simulink model "Waehrungsmodelle"  (R2014a)
settings: Solver=ode1  StartTime=0.0  StopTime=100  FixedStep=1  MaxStep=1  MinStep=1  RelTol=1e-3
(part 16 of 18)

== system Waehrungsmodelle/Währungssystem6/Populationsmodell ==
  note: Geburten
  Umweltqualität : Inport
  Dienstleistungsqualität : Inport  Port=2
  Güterangebotsqualität bei vorhandem Einkommen : Inport  Port=3
  Ausgleichsfaktor : Constant  Value=0.3
  Dienstleistungs- multiplikator : Sum
  Divide1 : Product  Inputs=*/
  Divide2 : Product  Inputs=*/
  Divide3 : Product  Inputs=*/
  Erwachsene : Sum  Inputs=+--
  Fertilitätsmultiplikator : Product  Inputs=4
  Fertilitätsrate pro Frau : Constant  Value=3/40
  Frauenanteil pro Erwachsene : Constant  Value=0.5
  Güterangebotsqualitäts- multiplikator : Sum
  Jahre der Altersklasse : Constant  Value=15
  Jahre der Altersklasse1 : Constant  Value=10
  Jahre der Altersklasse2 : Constant  Value=40
  Kinder : Sum  Inputs=+--
  Lebensqualitätsfaktor : Product  Inputs=/
  Product{,1..3} (4 alike) : Product  Inputs=3
  Schüler / Studenten : Sum  Inputs=+--
  Start Erwachsene: 55 : Integrator  InitialCondition=55
  Start Kinder: 13 : Integrator  InitialCondition=13
  Start Schüler: 11 : Integrator  InitialCondition=11
  Sterblichkeitsrate Kinder : Constant  Value=0.003
  Sterblichkeitsrate1 : Constant  Value=0.002
  Sterblichkeitsrate2 : Constant  Value=0.004
  Umwelt- multiplikator : Sum
  Erwerbsfähige : Outport
  wires:
  Product/1 -> Kinder/1
  Jahre der Altersklasse2/1 -> Divide3/2
  Jahre der Altersklasse/1 -> Divide1/2
  Divide1/1 -> Schüler / Studenten/1, Kinder/3
  Sterblichkeitsrate1/1 -> Product1/2
  Sterblichkeitsrate Kinder/1 -> Product2/2
  Divide2/1 -> Schüler / Studenten/3, Erwachsene/1
  Start Schüler: 11/1 -> Product1/3, Divide2/1
  Jahre der Altersklasse1/1 -> Divide2/2
  Sterblichkeitsrate2/1 -> Product3/2
  Start Erwachsene: 55/1 -> Erwerbsfähige/1, Product3/3, Divide3/1, Product/1
  Erwachsene/1 -> Start Erwachsene: 55/1
  Kinder/1 -> Start Kinder: 13/1
  Start Kinder: 13/1 -> Product2/3, Divide1/1
  Schüler / Studenten/1 -> Start Schüler: 11/1
  Ausgleichsfaktor/1 -> Umwelt- multiplikator/2, Güterangebotsqualitäts- multiplikator/1, Dienstleistungs- multiplikator/1
  Fertilitätsmultiplikator/1 -> Product/3
  Umweltqualität/1 -> Umwelt- multiplikator/1
  Dienstleistungs- multiplikator/1 -> Lebensqualitätsfaktor/1, Fertilitätsmultiplikator/4
  Fertilitätsrate pro Frau/1 -> Fertilitätsmultiplikator/1
  Umwelt- multiplikator/1 -> Fertilitätsmultiplikator/2
  Dienstleistungsqualität/1 -> Dienstleistungs- multiplikator/2
  Product2/1 -> Kinder/2
  Product1/1 -> Schüler / Studenten/2
  Divide3/1 -> Erwachsene/3
  Product3/1 -> Erwachsene/2
  Lebensqualitätsfaktor/1 -> Product3/1, Product1/1, Product2/1
  Güterangebotsqualität bei vorhandem Einkommen/1 -> Güterangebotsqualitäts- multiplikator/2
  Güterangebotsqualitäts- multiplikator/1 -> Fertilitätsmultiplikator/3
  Frauenanteil pro Erwachsene/1 -> Product/2

== system Waehrungsmodelle/Währungssystem6/Staat ==
  Kreditvergabe : Inport
  Kreditrückzahlung : Inport  Port=2
  Finanzbedarf Arbeitslosigkeit : Inport  Port=3
  Dienstleistungsqualität : Inport  Port=4
  Steuern Bank : Inport  Port=5
  Steuern Unternehmen : Inport  Port=6
  Rohstoffabgabe : Inport  Port=7
  Umweltqualität : Inport  Port=8
  MATLAB Function : MATLAB Function  TreatAsAtomicUnit=on
  Kreditbedarf : Outport
  Finanzierung Öffentlicher Dienstleistungen : Outport  Port=2
  Geldbestand Staat : Outport  Port=3
  Steuersatz : Outport  Port=4
  Ressourcen Steuer : Outport  Port=5
  wires:
  Steuern Unternehmen/1 -> MATLAB Function/6(SteuernUnternehmen)
  Dienstleistungsqualität/1 -> MATLAB Function/4(Dienstleistungsqualitaet)
  MATLAB Function/4(SteuersatzOut) -> Steuersatz/1
  MATLAB Function/2(FinanzierungOeffentlicheDienstleistungen) -> Finanzierung Öffentlicher Dienstleistungen/1
  Finanzbedarf Arbeitslosigkeit/1 -> MATLAB Function/3(FinanzbedarfArbeitslosigkeit)
  MATLAB Function/3(GeldbestandStaat) -> Geldbestand Staat/1
  Kreditrückzahlung/1 -> MATLAB Function/2(Kreditrueckzahlung)
  MATLAB Function/1(Kreditbedarf) -> Kreditbedarf/1
  Steuern Bank/1 -> MATLAB Function/5(SteuernBanken)
  Kreditvergabe/1 -> MATLAB Function/1(KreditvergabeNeuStaat)
  MATLAB Function/5(RessourcenAbgabesatzOut) -> Ressourcen Steuer/1
  Rohstoffabgabe/1 -> MATLAB Function/7(Rohstoffabgabe)
  Umweltqualität/1 -> MATLAB Function/8(Umweltqualitaet)

== system Waehrungsmodelle/Währungssystem6/Umwelt ==
  Ressourcenbedarf : Inport
  Umwelt : MATLAB Function  TreatAsAtomicUnit=on
  abgebaute Ressourcen : Outport
  verhandene Ressourcen : Outport  Port=2
  Umweltqualität : Outport  Port=3
  wires:
  Umwelt/3(Umweltqualitaet) -> Umweltqualität/1
  Umwelt/2(VorhandeneRessourcenOut) -> verhandene Ressourcen/1
  Umwelt/1(AbgebauteRessourcen) -> abgebaute Ressourcen/1
  Ressourcenbedarf/1 -> Umwelt/1(Ressourcenbedarf)

== system Waehrungsmodelle/Währungssystem6/Unternehmen ==
  Erwerbsfähige : Inport
  Neue Kreditvergabe der Unternehmen : Inport  Port=2
  Kreditrückzahlung der Unternehmen : Inport  Port=3
  Rohstoffe : Inport  Port=4
  Güterkonsum Inland : Inport  Port=5
  Güterkonsum Ausland : Inport  Port=6
  RessourcenAbgabe Steuersatz : Inport  Port=7
  Kreditzinssatz Inland : Inport  Port=8
  Kreditzinssatz Ausland : Inport  Port=9
  Steuersatz : Inport  Port=10
  Neue Kreditvergabe der Unternehmen Ausland : Inport  Port=11
  Kreditrückzahlung der Unternehmen Ausland : Inport  Port=12
  MATLAB Function : MATLAB Function  TreatAsAtomicUnit=on
  Inflation : Outport
  Rohstoffbedarf : Outport  Port=2
  Arbeitsplätze der Unternehmen : Outport  Port=3
  Güterangebot Inland : Outport  Port=4
  Arbeitslohn : Outport  Port=5
  zukünftiger Arbeitsdarf der Unternehmen : Outport  Port=6
  Güterpreis : Outport  Port=7
  Steuern von Unternehmen : Outport  Port=8
  Rohstoffabgabe : Outport  Port=9
  Kreditbedarf Inland : Outport  Port=10
  Kreditbedarf Ausland : Outport  Port=11
  Technischer Fortschritt Rationalität : Outport  Port=12
  Technischer Fortschritt Ressourcen : Outport  Port=13
  Wirtschaftswachstum : Outport  Port=14
  Güterangebot Ausland : Outport  Port=15
  wires:
  MATLAB Function/8(SteuernUnternehmen) -> Steuern von Unternehmen/1
  MATLAB Function/7(GueterpreisOut) -> Güterpreis/1
  Neue Kreditvergabe der Unternehmen/1 -> MATLAB Function/2(NeueKreditvergabeUnternehmen)
  Kreditrückzahlung der Unternehmen/1 -> MATLAB Function/3(KreditrueckzahlungUnternehmen)
  MATLAB Function/6(BenoetigterArbeitsbedarfUnternehmen) -> zukünftiger Arbeitsdarf der Unternehmen/1
  MATLAB Function/4(GueterangebotInland) -> Güterangebot Inland/1
  MATLAB Function/5(ArbeitslohnOut) -> Arbeitslohn/1
  MATLAB Function/2(Rohstoffbedarf) -> Rohstoffbedarf/1
  MATLAB Function/1(Inflation) -> Inflation/1
  Erwerbsfähige/1 -> MATLAB Function/1(Erwerbsfaehige)
  MATLAB Function/3(ArbeitsplaetzeUnternehmen) -> Arbeitsplätze der Unternehmen/1
  Rohstoffe/1 -> MATLAB Function/4(Rohstoffe)
  Güterkonsum Inland/1 -> MATLAB Function/5(GueterkonsumInland)
  MATLAB Function/9(RessourcenAbgabeSteuer) -> Rohstoffabgabe/1
  MATLAB Function/11(KreditbedarfAusland) -> Kreditbedarf Ausland/1
  MATLAB Function/12(TechnischeVerbesserungRationalitaetOut) -> Technischer Fortschritt Rationalität/1
  MATLAB Function/13(TechnischeVerbesserungRessourcenOut) -> Technischer Fortschritt Ressourcen/1
  Güterkonsum Ausland/1 -> MATLAB Function/6(GueterkonsumAusland)
  RessourcenAbgabe Steuersatz/1 -> MATLAB Function/7(RessourcenAbgabeSteuersatz)
  Kreditzinssatz Inland/1 -> MATLAB Function/8(KreditZinssatzInland)
  Kreditzinssatz Ausland/1 -> MATLAB Function/9(KreditZinssatzAusland)
  Steuersatz/1 -> MATLAB Function/10(Steuersatz)
  MATLAB Function/10(KreditbedarfInland) -> Kreditbedarf Inland/1
  MATLAB Function/14(Wirtschaftswachstum) -> Wirtschaftswachstum/1
  MATLAB Function/15(GueterangebotAusland) -> Güterangebot Ausland/1
  Neue Kreditvergabe der Unternehmen Ausland/1 -> MATLAB Function/11(NeueKreditvergabeUnternehmenAusland)
  Kreditrückzahlung der Unternehmen Ausland/1 -> MATLAB Function/12(KreditrueckzahlungUnternehmenAusland)

== system Waehrungsmodelle/Währungssystem6/Wechselkursberechnung ==
  Güterpreis Ausland : Inport
  Güterkonsum im Inland von Gütern vom Ausland : Inport  Port=2
  Güterkonsum im Ausland von Gütern im Inland : Inport  Port=3
  MATLAB Function : MATLAB Function  TreatAsAtomicUnit=on
  Güterpreis Ausland in Eigenwährung : Outport
  Wechselkursfaktor : Outport  Port=2
  Gesamter Güterkonsum im Ausland von Gütern im Inland : Outport  Port=3
  Gesamter Güterkonsum im Inland von Gütern vom Ausland : Outport  Port=4
  wires:
  Güterpreis Ausland/1 -> MATLAB Function/1(GueterpreisAusland)
  Güterkonsum im Inland von Gütern vom Ausland/1 -> MATLAB Function/2(GueterKonsumImInlandVomAusland)
  Güterkonsum im Ausland von Gütern im Inland/1 -> MATLAB Function/3(GueterKonsumImAuslandVomInland)
  MATLAB Function/1(GueterpreisAuslandInEigenwaehrung) -> Güterpreis Ausland in Eigenwährung/1
  MATLAB Function/2(Wechselkursfaktor) -> Wechselkursfaktor/1
  MATLAB Function/3(GesamterGueterKonsumImAuslandVomInlandOut) -> Gesamter Güterkonsum im Ausland von Gütern im Inland/1
  MATLAB Function/4(GesamterGueterKonsumImInlandVomAuslandOut) -> Gesamter Güterkonsum im Inland von Gütern vom Ausland/1

== system Waehrungsmodelle/Währungssystem6/Öffentliche Dienstleistungen ==
  Finanzierung : Inport
  Erwerbsfähige : Inport  Port=2
  Arbeitslohn : Inport  Port=3
  MATLAB Function : MATLAB Function  TreatAsAtomicUnit=on
  Arbeitsplätze Dienstleistung : Outport
  Dienstleistungsqualität : Outport  Port=2
  wires:
  Arbeitslohn/1 -> MATLAB Function/3(Arbeitslohn)
  Erwerbsfähige/1 -> MATLAB Function/2(Erwerbsfaehige)
  Finanzierung/1 -> MATLAB Function/1(Finanzierung)
  MATLAB Function/1(ArbeitsplaetzeDienstleistung) -> Arbeitsplätze Dienstleistung/1
  MATLAB Function/2(Dienstleistungsqualitaet) -> Dienstleistungsqualität/1

== matlab function Waehrungsmodelle/Währungssystem1/Haushalte/MATLAB Function ==
  data: Erwerbsfaehige input; GueterkonsumInland output; ArbeitsplaetzeDienstleistungen input; ArbeitsplaetzeUnternehmen input; NeueKreditvergabeInland input; KreditrueckzahlungInland input; GueterAngebotInland input; Arbeitslohn input; GueterpreisInland input; FinanzierungArbeitslosigkeit output; Spareinlagen output; KreditbedarfInland output; ArbeiterUnternehmen output; GueterVorratHaushalte output; GueterangebotsqualitaetOut output; Arbeitslosenquote output; GueterpreisAusland input; GueterkonsumAusland output; KreditbedarfAusland output; NeueKreditvergabeAusland input; KreditrueckzahlungAusland input; GueterAngebotAusland input; KreditZinssatzInland input; KreditZinssatzAusland input
function [GueterkonsumInland, FinanzierungArbeitslosigkeit, Spareinlagen, KreditbedarfInland, ...
              ArbeiterUnternehmen, GueterVorratHaushalte, GueterangebotsqualitaetOut, ...
              Arbeitslosenquote, GueterkonsumAusland, KreditbedarfAusland] = ...
    Haushalte(Erwerbsfaehige, ArbeitsplaetzeDienstleistungen, ArbeitsplaetzeUnternehmen, ...
            NeueKreditvergabeInland, KreditrueckzahlungInland, GueterAngebotInland, Arbeitslohn, ...
            GueterpreisInland, GueterpreisAusland, NeueKreditvergabeAusland, ...
            KreditrueckzahlungAusland, GueterAngebotAusland, KreditZinssatzInland, KreditZinssatzAusland)
 %# Submodul zur Berechnung der Abläufe bzgl. der Haushalte
 
% Es wird eine Gütereinheit pro Zeiteinheit und Erwerbsfaehiger
% verbraucht;
persistent GueterVorrat;

% Angebotsqualität der Güter [0 - 1]
% Werden weniger Güter angeboten als benötigt oder ist die Anzahl der 
% benötigten Güter nicht mehr bezahlbar sinkt die Qualität
persistent Gueterangebotsqualitaet;

    % Anfangsvorrat
    if isempty(GueterVorrat)
       GueterVorrat = 100;
    end 
    
    if isempty(Gueterangebotsqualitaet)
       Gueterangebotsqualitaet = 1;
    end     
    
    % Beschäftigte bei Öffentlichen Dienstleistungen bekommen 80 % vom
    % Lohnniveau der Unternehmen
    Dienstleistungslohnfaktor = 0.8;
    
    % Arbeitslose bekommen vom Staat 50% des Lohnnivaus
    Arbeitslosenlohnfaktor = 0.5;    
    
    % Maximale Vorratszeit
    MaximaleVorratszeit = 4;
    
    % Der maximale Vorrat gilt für 4 Zeiteinheiten
    MaximalerVorrat = Erwerbsfaehige * MaximaleVorratszeit; 
    
    
    % Gueterverbrauch pro Zeiteinheit
    GueterVorrat = GueterVorrat -  Erwerbsfaehige;    

    if GueterVorrat <= 0
         % Sind weniger Vorräte als fuer eine Zeiteinheit vorhanden, 
         % sinkt die Güterqualität
        Gueterangebotsqualitaet = Gueterangebotsqualitaet - 0.1;
        Gueterangebotsqualitaet = max(Gueterangebotsqualitaet, 0);
    else 
         % Sind mehr Vorräte als fuer eine Zeiteinheit vorhanden, 
         % steigt die Güterqualität        
        Gueterangebotsqualitaet = Gueterangebotsqualitaet + 0.1;
        Gueterangebotsqualitaet = min(Gueterangebotsqualitaet, 1);        
    end       
    
    GueterangebotsqualitaetOut = Gueterangebotsqualitaet;  
    
    % Es können maximal die vergleibenden Erwerbsfähigen oder der
    % notwendige Arbeiterbedarf eingesetzt werden
    ArbeiterUnternehmen = Erwerbsfaehige - ArbeitsplaetzeDienstleistungen;
    
    % die Arbeitslosen sind alle Erwerbsfähigen, welche keinen Arbeitsplatz
    % haben
    Arbeitslose = Erwerbsfaehige - (ArbeitsplaetzeUnternehmen + ArbeitsplaetzeDienstleistungen );
    % Arbeitslosenquote [0 - 1]
    % Auf Grund von Rundungen kann die Arbeitslosenquote min. 0 sein.
    Arbeitslosenquote = max(0, Arbeitslose / Erwerbsfaehige);
    
   
    
    % Einkommensberechnung für die Arbeitsplätze bei Unternehmen
    EinkommenUnternehmen = ArbeitsplaetzeUnternehmen * Arbeitslohn ;
    
    % Einkommensberechnung für die Arbeitsplätze bei Öffentlichen Dienstleistungen
    EinkommenDienstleistungen = ArbeitsplaetzeDienstleistungen * Arbeitslohn * Dienstleistungslohnfaktor;
    
    % Finanzierungsbedarf fuer Arbeitslosigkeit
    EinkommenArbeitslosigkeit = Arbeitslose * Arbeitslohn * Arbeitslosenlohnfaktor;
    FinanzierungArbeitslosigkeit = EinkommenArbeitslosigkeit;
    
    % Berechnung des Gesamteinkommens
    Gesamteinkommen = EinkommenUnternehmen + EinkommenDienstleistungen + EinkommenArbeitslosigkeit;           
        
    % Genehmigung der letzten Kreditanfrage
    Gesamteinkommen = Gesamteinkommen + NeueKreditvergabeInland + NeueKreditvergabeAusland;   
    
    % Rückzahlung der offenen Kreditrate
    Gesamteinkommen = Gesamteinkommen - KreditrueckzahlungInland - KreditrueckzahlungAusland;    
    
    % Prüfen welche Güter die günstigeren sind (Inlandsgüter oder
    % Auslandsgüter)
    if GueterpreisInland <= GueterpreisAusland
        % Wenn die Güter im Inland günstiger sind
        
        % Güter nachkaufen solange das Geld reicht oder das Vorratsmaximum erreicht
        % wurde, in Abhängigkeit des Güterangebots
        MoeglicheGueternachfrage = floor(Gesamteinkommen / GueterpreisInland);      
        % Die kleinste Gueternachfrage ist immer 50% des normalen
        % Verbrauchs der Güter
        GueterkonsumInland = max(0, min(MoeglicheGueternachfrage, GueterAngebotInland));

        % Wenn genug Güter auf Vorrat Komsum auf 50% senken
        if GueterVorrat > MaximalerVorrat
            GueterkonsumInland = GueterkonsumInland / 2;    
        end

        GueterVorrat = GueterVorrat + GueterkonsumInland;
        UebrigesGueterangebot = GueterAngebotInland - GueterkonsumInland;
        UebrigesEinkommen = Gesamteinkommen - (GueterkonsumInland * GueterpreisInland);  

        % Wenn noch Geld übrig ist und genug Geld vorhanden im Ausland die
        % Güter kaufen
        if GueterVorrat < MaximalerVorrat && UebrigesEinkommen > 0
            % Güter nachkaufen solange das Geld reicht oder das Vorratsmaximum erreicht
            % wurde, in Abhängigkeit des Güterangebots
            MoeglicheGueternachfrageAusland = floor(UebrigesEinkommen / GueterpreisAusland);              
            GueterkonsumAusland = max(0, min(min(MoeglicheGueternachfrageAusland, GueterAngebotAusland), MaximalerVorrat-GueterVorrat));           
            
            GueterVorrat = GueterVorrat + GueterkonsumAusland;
            UebrigesEinkommen = UebrigesEinkommen - (GueterkonsumAusland * GueterpreisAusland);                  
        else
            GueterkonsumAusland = 0;
        end        
    else
        % Wenn die Güter im Ausland günstiger sind
        
        % Güter nachkaufen solange das Geld reicht oder das Vorratsmaximum erreicht
        % wurde, in Abhängigkeit des Güterangebots
        % Es können maximal 50% der Güter aus dem Ausland gekauft werden
        MoeglicheGueternachfrage = min(0, min(Erwerbsfaehige/2, floor(Gesamteinkommen / GueterpreisAusland)));    

        GueterkonsumAusland = max(0, min(MoeglicheGueternachfrage, GueterAngebotAusland));

        % Wenn genug Güter auf Vorrat Komsum auf 50% senken
        if GueterVorrat > MaximalerVorrat
            GueterkonsumAusland = GueterkonsumAusland / 2;    
        end

        GueterVorrat = GueterVorrat + GueterkonsumAusland;

        UebrigesEinkommen = Gesamteinkommen - (GueterkonsumAusland * GueterpreisAusland);  

        % Wenn noch Geld übrig ist und genug Geld vorhanden im Ausland die
        % Güter kaufen
        if GueterVorrat < MaximalerVorrat && UebrigesEinkommen > 0
            % Güter nachkaufen solange das Geld reicht oder das Vorratsmaximum erreicht
            % wurde, in Abhängigkeit des Güterangebots
            MoeglicheGueternachfrageInland = floor(UebrigesEinkommen / GueterpreisInland);              
            GueterkonsumInland = max(0, min(MoeglicheGueternachfrageInland, GueterAngebotInland));                       
            GueterkonsumInland = GueterkonsumInland * min(0, 1.5 - GueterVorrat / MaximalerVorrat);
            
            GueterVorrat = GueterVorrat + GueterkonsumInland;
            UebrigesGueterangebot = GueterAngebotInland - GueterkonsumInland;
            UebrigesEinkommen = UebrigesEinkommen - (GueterkonsumInland * GueterpreisInland);                  
        else
            GueterkonsumInland = 0;
            UebrigesGueterangebot = 0;
        end            
    end   
    
    
    % Prüfung ob ein Kredit notwendig ist, da noch zu wenig Güter gekauft
    % wurden und Güter vorhanden sind
    if GueterVorrat < Erwerbsfaehige *2 && UebrigesGueterangebot > 0
        % Berechnung der notwendigen Güter bis zur nächsten Zeiteinheit
        BenoetigteGueter = Erwerbsfaehige;                
                        
        % Berechnung des Kreditbedarfs
        Kreditbedarf = BenoetigteGueter * GueterpreisInland;  
        % Kreditbedarf auf In- und Ausland aufteilen
        % Der Kredit mit dem geringeren Zinssatz wird bevorzugt und 70%
        % verwendet. Der teurere Kredit wird mit 30% verwendet.
        if KreditZinssatzInland <= KreditZinssatzAusland
            KreditbedarfInland = Kreditbedarf * 0.7;
            KreditbedarfAusland = Kreditbedarf * 0.3;
        else
            KreditbedarfAusland = Kreditbedarf * 0.7;
            KreditbedarfInland = Kreditbedarf * 0.3;        
        end        
    else
        % Kein Kreditbedarf
        KreditbedarfInland = 0;        
        KreditbedarfAusland = 0;  
    end
    
    % Übriges Geld sparen
    Spareinlagen = UebrigesEinkommen;
    
    GueterVorratHaushalte = GueterVorrat;

== matlab function Waehrungsmodelle/Währungssystem1/Öffentliche Dienstleistungen/MATLAB Function ==
  data: Finanzierung input; ArbeitsplaetzeDienstleistung output; Erwerbsfaehige input; Arbeitslohn input; Dienstleistungsqualitaet output
function [ArbeitsplaetzeDienstleistung, Dienstleistungsqualitaet] = OeffentlicheDienstleistungen(Finanzierung, Erwerbsfaehige, Arbeitslohn)
%# Submodul zur Berechnung das Öffentliche Dienstleistungsmodell

    persistent Arbeitsplaetze;

    % Anfangsarbeitsplätze
    if isempty(Arbeitsplaetze)
       Arbeitsplaetze = 20;
    end 

    % Da der Arbeitslohn ein Referenzlohn der privaten Unternehmen ist wird
    % dieser angepasst und um 20 % gesenkt
    LohnNiveauOeffentlicherDienst = 0.8;
    Arbeitslohn = Arbeitslohn * LohnNiveauOeffentlicherDienst;
    
    % Es können nicht mehr Arbeitsplätze wie Erwerbsfähige vorhanden sind
    % besetzt werden
    if Erwerbsfaehige < Arbeitsplaetze
        Arbeitsplaetze = Erwerbsfaehige;
    end

    % Existiert nicht genug Geld für die öffentlichen Dientleistungen
    % werden die Arbeitsplätze an die Finanzierung vom Staat angepasst.
    if (Finanzierung < Arbeitsplaetze * Arbeitslohn)
        Arbeitsplaetze = floor(Finanzierung / Arbeitslohn);        
    end          
       
    ArbeitsplaetzeDienstleistung = Arbeitsplaetze;
    
    % Berechnet Dienstleistungsqualitaet mit min:0.2 und max:1
    % indem die Arbeitsplätze der öffentlichen Dienstleistungen durch die
    % gesamten Erwerbstätigen geteilt werden und als Ausgleichfaktor mit drei
    % multipliziert wird. Somit ist es optimal wenn min. 1/3 aller
    % Erwerbsfähigen bei den öffentlichen Dienstleistungen arbeiten
    Dienstleistungsqualitaet = max(0.2, min(1, 3 * Arbeitsplaetze / Erwerbsfaehige));

== matlab function Waehrungsmodelle/Währungssystem1/Banken/MATLAB Function ==
  data: EinlagenAenderungHaushalte input; KreditbedarfHaushalte input; KreditbedarfUnternehmen input; KreditbedarfHaushalteAusland input; KreditbedarfUnternehmenAusland input; KreditbedarfStaat input; Steuersatz input; Leitzins input; Mindestreservesatz input; MaximaleNotenbankGeldmenge input; KontoHaushalteOut output; KrediteHaushalteOut output; KrediteUnternehmenOut output; KrediteStaatOut output; KreditvergabeHaushalte output; KreditvergabeUnternehmen output; KreditvergabeStaat output; KreditrueckzahlungHaushalte output; KreditrueckzahlungUnternehmen output; KreditrueckzahlungStaat output; BankgewinnNachSteuern output; BankenSteuern output; BankKontostand output; Bankenzinssatz output; KrediteUnternehmenAuslandOut output; KreditrueckzahlungUnternehmenAusland output; KreditvergabeUnternehmenAusland output; KrediteHaushalteAuslandOut output; KreditrueckzahlungHaushalteAusland output; KreditvergabeHaushalteAusland output
function [KontoHaushalteOut, KrediteHaushalteOut, KrediteUnternehmenOut, KrediteStaatOut, ... 
            KreditvergabeHaushalte, KreditvergabeUnternehmen, KreditvergabeStaat, ...
            KreditrueckzahlungHaushalte, KreditrueckzahlungUnternehmen, KreditrueckzahlungStaat, ...
            BankgewinnNachSteuern, BankenSteuern, BankKontostand, Bankenzinssatz, ...
            KrediteUnternehmenAuslandOut, KreditrueckzahlungUnternehmenAusland, KreditvergabeUnternehmenAusland, ...
            KrediteHaushalteAuslandOut, KreditrueckzahlungHaushalteAusland, KreditvergabeHaushalteAusland] = ...
    Banken(EinlagenAenderungHaushalte, KreditbedarfHaushalte, KreditbedarfUnternehmen, ...
            KreditbedarfHaushalteAusland, KreditbedarfUnternehmenAusland, KreditbedarfStaat, ...
            Steuersatz, Leitzins, Mindestreservesatz, MaximaleNotenbankGeldmenge)
% Submodell Banken zur Berechnung der Geld-Prozesse zwischen 
% Banken und Haushalten

% ANMERKUNG:
% Warum gibt es auf der einen Seite Kredite und Guthaben der Haushalte?
% Der überwigende Teil der Geldes MUSS den Haushalten gehören, da diese
% die Unternehmen und Banken besitzen. Ich vermute, dass es in einen
% demokratischen Staat nicht möglich ist, dass der Staat mehr Geld als 
% die Bevölkerung besitzt.
% Die ungleiche Geldverteilung ist dafür verantwortlich, dass die Haushalte
% auf der einen Seite Spareinlagen und Kredite haben. Ohne Spareinlagen wäre
% es aktuell nicht möglich Kredite überhaupt zu vergeben.

% Der Zinsspread ist die Prozentuale-Differenz der Zinsweitergabe bei
% Krediten und Anlagen
persistent Zinsspread;

% interner Zinssatz
persistent InternerZinssatz;

% aktuelle Kredithöhe der Unternehmen
persistent KrediteUnternehmen;

% aktuelle Kredithöhe des Staats
persistent KrediteStaat;

% aktuelle Kredithöhe der Haushalte
persistent KrediteHaushalte;

% aktuelle Kredithöhe der Unternehmen im Ausland
persistent KrediteUnternehmenAusland;

% aktuelle Kredithöhe der Haushalte im Ausland
persistent KrediteHaushalteAusland;

% aktueller Kontostand der Haushalte
persistent KontoHaushalte;

% Rückzahlungsdauer des Kredits
persistent Kreditrueckzahlungsdauer;

% Vermnögen der Bank aus den Gewinnen
persistent KontoBank;

    % Zinsspread 1%
    if isempty(Zinsspread)
       Zinsspread = 0.01;
    end 
    
    % interner Zinssatz auf den Leitzins festlegen
    if isempty(InternerZinssatz)
       InternerZinssatz = Leitzins;
    end     
    
    % Rückzahlungsdauer 15 Zeiteinheiten
    if isempty(Kreditrueckzahlungsdauer)
       Kreditrueckzahlungsdauer = 15;
    end     
   
    if isempty(KontoBank)
       KontoBank = 400;
    end   
    if isempty(KontoHaushalte)
       KontoHaushalte = 0;
    end   
    if isempty(KrediteHaushalte)
       KrediteHaushalte = 200;
    end     
    if isempty(KrediteUnternehmen)
       KrediteUnternehmen = 200;
    end 
    if isempty(KrediteStaat)
       KrediteStaat = 200;
    end     
    if isempty(KrediteUnternehmenAusland)
       KrediteUnternehmenAusland = 200;
    end     
    if isempty(KrediteHaushalteAusland)
       KrediteHaushalteAusland = 200;
    end   
    
    % Habenzinsen berechnen
    HabenZinsen = KontoHaushalte * (InternerZinssatz - Zinsspread);
    KontoHaushalte = KontoHaushalte + HabenZinsen;
    
    % Ein- / Auszahlung
    KontoHaushalte = KontoHaushalte + EinlagenAenderungHaushalte;    
      
    % Maximale Kreditvergabe anhand des Mindestreservesatzes und der 
    % Spareinlagen der Haushalte
    MaximaleKreditvergabe = KontoHaushalte * (1 / Mindestreservesatz); 

    % Maximale Geldmenge, welche von der Notenbank zur Verfügung gestellt wird
    % Prüfung anhand der Maximalen Kreditvergabe, da Guthaben = Kredit    
    MaximaleKreditvergabe = max(MaximaleNotenbankGeldmenge, MaximaleKreditvergabe);
    
    Gesamtkredit = KrediteHaushalte + KrediteUnternehmen + KrediteStaat;
    MaximaleKreditvergabe = MaximaleKreditvergabe - Gesamtkredit;

    % Wenn genug Geld auf dem Konto ist, so wird ein prozenualer Anteil mit
    % dem neuen Kreditbedarf verrechnet ==> 10 %    
    if KontoHaushalte > KreditbedarfHaushalte && KreditbedarfHaushalte > 0
       AusgleichbarerGeldBedarf = KreditbedarfHaushalte * 0.1;
       KontoHaushalte = KontoHaushalte - AusgleichbarerGeldBedarf;
       KreditbedarfHaushalte = KreditbedarfHaushalte - AusgleichbarerGeldBedarf;
    end         

    % Kreditberechnung für Haushalte      
    [KrediteHaushalte, KreditvergabeHaushalte, KreditrueckzahlungHaushalte, ...
                        SollZinsenHaushalte, MaximaleKreditvergabe] = ...
        Kreditberechnung(KrediteHaushalte, KreditbedarfHaushalte, MaximaleKreditvergabe, ...
                        InternerZinssatz, Zinsspread, Kreditrueckzahlungsdauer);                    
    
    % Kreditberechnung für Staat   
    [KrediteStaat, KreditvergabeStaat, KreditrueckzahlungStaat, SollZinsenStaat, ...
                        MaximaleKreditvergabe] = ...
        Kreditberechnung(KrediteStaat, KreditbedarfStaat, MaximaleKreditvergabe, ...
                        InternerZinssatz, Zinsspread, Kreditrueckzahlungsdauer);                    

    % Kreditberechnung für Unternehmen   
    [KrediteUnternehmen, KreditvergabeUnternehmen, KreditrueckzahlungUnternehmen, ...
                        SollZinsenUnternehmen, MaximaleKreditvergabe] = ...
        Kreditberechnung(KrediteUnternehmen, KreditbedarfUnternehmen, MaximaleKreditvergabe, ...
                        InternerZinssatz, Zinsspread, Kreditrueckzahlungsdauer);

    % Kreditberechnung für Haushalte im Ausland
    [KrediteHaushalteAusland, KreditvergabeHaushalteAusland, KreditrueckzahlungHaushalteAusland, ...
                        SollZinsenHaushalteAusland, MaximaleKreditvergabe] = ...
        Kreditberechnung(KrediteHaushalteAusland, KreditbedarfHaushalteAusland, MaximaleKreditvergabe, ...
                        InternerZinssatz, Zinsspread, Kreditrueckzahlungsdauer);                                        

    % Kreditberechnung für Unternehmen im Ausland
    [KrediteUnternehmenAusland, KreditvergabeUnternehmenAusland, KreditrueckzahlungUnternehmenAusland, ...
                        SollZinsenUnternehmenAusland, MaximaleKreditvergabe] = ...
        Kreditberechnung(KrediteUnternehmenAusland, KreditbedarfUnternehmenAusland, MaximaleKreditvergabe, ...
                        InternerZinssatz, Zinsspread, Kreditrueckzahlungsdauer);                    
                    
    % Berechnung der Notenbankkredite
    NotenbankKredite = (KrediteHaushalte + KrediteUnternehmen + KrediteStaat + ...
                    KrediteHaushalteAusland + KrediteUnternehmenAusland) - (KontoBank + KontoHaushalte);
    NotenbankKredite = max(NotenbankKredite, 0);
    NotenbankZinsen = NotenbankKredite * Leitzins;
    KontoBank = KontoBank - NotenbankZinsen;   
    
    % Gewinnberechnung der Bank
    SollZinsen = SollZinsenHaushalte + SollZinsenStaat + SollZinsenUnternehmen ...
                + SollZinsenHaushalteAusland + SollZinsenUnternehmenAusland;
    Bankgewinn = SollZinsen - HabenZinsen;
    
    % Steuerberechnung der Bank
    BankenSteuern = max(Bankgewinn * Steuersatz, 0);
    BankgewinnNachSteuern = Bankgewinn - BankenSteuern;
    
    % Kontostand der Bank berechnen
    KontoBank = KontoBank + Bankgewinn - BankenSteuern;
    
    % Zinssätze anpassen (Zinsänderung anpassen y = -0.00005x + 0.001;
    Zinsaenderung = -0.00005 * BankgewinnNachSteuern + 0.001;
    InternerZinssatz = InternerZinssatz + Zinsaenderung;
    
    KrediteStaatOut = KrediteStaat;
    KrediteUnternehmenOut = KrediteUnternehmen;
    KrediteHaushalteOut = KrediteHaushalte;
    KrediteUnternehmenAuslandOut = KrediteUnternehmenAusland;
    KrediteHaushalteAuslandOut = KrediteHaushalteAusland;    
    KontoHaushalteOut = KontoHaushalte;    
    BankKontostand = KontoBank;
    Bankenzinssatz = InternerZinssatz;

== matlab function Waehrungsmodelle/Währungssystem1/Staat/MATLAB Function ==
  data: KreditvergabeNeuStaat input; Kreditrueckzahlung input; FinanzbedarfArbeitslosigkeit input; Dienstleistungsqualitaet input; Kreditbedarf output; SteuernBanken input; SteuernUnternehmen input; Rohstoffabgabe input; FinanzierungOeffentlicheDienstleistungen output; GeldbestandStaat output; SteuersatzOut output; RessourcenAbgabesatzOut output; Umweltqualitaet input
function [Kreditbedarf, FinanzierungOeffentlicheDienstleistungen, GeldbestandStaat, ...
            SteuersatzOut, RessourcenAbgabesatzOut] = ...
    Staat(KreditvergabeNeuStaat, Kreditrueckzahlung, FinanzbedarfArbeitslosigkeit, ...
            Dienstleistungsqualitaet, SteuernBanken, SteuernUnternehmen, Rohstoffabgabe, Umweltqualitaet)
%# Submodul zur Berechnung der Staatsprozesse

    % Geldbestand
    persistent Geldbestand;    

    % letzte Finanzierung
    persistent LetzteFinanzierung;
    
    % Steuersatz in Prozent
    persistent Steuersatz;  
    
    % Ressourcenabgabesatz
    persistent RessourcenAbgabesatz;
    
    % Geldbestand
    if isempty(Geldbestand)
       Geldbestand = 100;
    end 
    % letzte Finanzierung
    if isempty(LetzteFinanzierung)
       LetzteFinanzierung = 30;
    end 
    % Steuersatz in Prozent
    if isempty(Steuersatz)
       Steuersatz = 0.4;
    end     
    % Ressourcenabgabesatz
    if isempty(RessourcenAbgabesatz)
       RessourcenAbgabesatz = 0.6;
    end       
    
    % Maximaler Steuersatz
    MaximalerSteuersatz = 0.6;
    
    % Steuereinkommen
    Steuereinkommen = SteuernBanken + SteuernUnternehmen + Rohstoffabgabe;
    
    % Abzug Kosten für Arbeitslose und Kreditrueckzahlung
    Steuereinkommen = Steuereinkommen  - (Kreditrueckzahlung + FinanzbedarfArbeitslosigkeit);
    
    % Aktuallisierung des Geldbestands
    Geldbestand = Geldbestand + Steuereinkommen + KreditvergabeNeuStaat;
    
    % Prüfen des Finanzierungsbedarfs
    if Dienstleistungsqualitaet > 0.9
        Finanzierungsbedarf = LetzteFinanzierung;        
    elseif Dienstleistungsqualitaet < 0.4
        Finanzierungsbedarf = LetzteFinanzierung * 1.05+5;   
    elseif Dienstleistungsqualitaet < 0.7
        Finanzierungsbedarf = LetzteFinanzierung * 1.02;           
    else
        Finanzierungsbedarf = LetzteFinanzierung * 1.01;        
    end                 

    Kreditbedarf = 0;
    % Prüfen ob der Steuersatz geändert werden sollte
    if Geldbestand > 150
        Steuersatz = max(0, Steuersatz - 0.01);   
    else
        Steuersatz = min(MaximalerSteuersatz, Steuersatz + 0.01);        
        Finanzierungsbedarf = LetzteFinanzierung * 0.9;
        % Wenn wenig Geld vorhanden ist, Kredit beantragen
        Kreditbedarf = (FinanzbedarfArbeitslosigkeit + Finanzierungsbedarf + 10) - Steuereinkommen;  
    end                
    
    FinanzierungOeffentlicheDienstleistungen = Finanzierungsbedarf;
    
    % Abgaben der Ressourcenabgabe berechnen
    if (Umweltqualitaet < 0.5)
        RessourcenAbgabesatz = RessourcenAbgabesatz + 0.02;    
    elseif (Umweltqualitaet < 0.7)
        RessourcenAbgabesatz = RessourcenAbgabesatz + 0.01;
    elseif (Umweltqualitaet > 0.9)
        RessourcenAbgabesatz = RessourcenAbgabesatz - 0.01;
    end
    
    % Kosten vom Geldbestand abziehen
    Geldbestand  = Geldbestand - FinanzierungOeffentlicheDienstleistungen;
       
    % Speichern der Werte
    LetzteFinanzierung = FinanzierungOeffentlicheDienstleistungen;
    SteuersatzOut = Steuersatz;
    GeldbestandStaat = Geldbestand;
    RessourcenAbgabesatzOut = RessourcenAbgabesatz;

== matlab function Waehrungsmodelle/Währungssystem1/Notenbank/MATLAB Function ==
  data: Gesamtkredite input; LeitzinsOut output; MindestreservesatzOut output; MaximaleNotenbankGeldmengeOut output; Arbeitslosenquote input; Inflation input; Wirtschaftswachtsum input
function [LeitzinsOut, MindestreservesatzOut, MaximaleNotenbankGeldmengeOut] = ...
    Notenbank(Gesamtkredite, Arbeitslosenquote, Inflation, Wirtschaftswachtsum)
%# Submodul zur Berechnung der Notenbankprozesse

% Leitzins der Notenbank => 0.03
persistent Leitzins;

% Mindestreservesatz => 0.01
persistent Mindestreservesatz;    

% Maximale Geldmenge, welche von der Notenbank vergeben werden kann
persistent MaximaleNotenbankGeldmenge;   

% festgelegter Geldmengenwachstum => 0.05
% Dieser Wert ist bei gedeckten Währungssystemen notwendig, da hiermit die
% Geldmenge mit dem Gesamtwert des Deckungswerts mitwachsen kann
Geldmengenwachstum = 0.05;

% gewünschte Inflation => 0.02
Inflationsziel = 0.02;

% Inflationstoleranz => 0.02
Inflationstoleranz = 0.02;

% Arbeitslosentoleranzquote => 0.08
Arbeitslosentoleranzquote = 0.08;

% Änderung des Leitzins
Leitzinsaenderung = 0;

    if isempty(Leitzins)
       Leitzins = 0.03;
    end  
    if isempty(Mindestreservesatz)
       Mindestreservesatz = 0.01;
    end  
    if isempty(MaximaleNotenbankGeldmenge)
       MaximaleNotenbankGeldmenge =  1000;
    end       
    
    % Pürfen, ob ein erlaubter Geldmengenwachstum sinnvoll ist
    if Gesamtkredite > MaximaleNotenbankGeldmenge * 0.9
        MaximaleNotenbankGeldmenge = MaximaleNotenbankGeldmenge * (1 + Geldmengenwachstum);
    end
    
    % Wenn das Wirtschaftswachtsum zu gering ist, wird der Leitzins gesenkt
    if Wirtschaftswachtsum < Leitzins
        Leitzinsaenderung = -0.001;
    else
        Leitzinsaenderung = 0.001;
    end
    
    % Wenn die Arbeitslosigkeit unter der Arbeitslosentoleranzquote ist, wird kann der Leitzins erhöht
    % sonst wird der Leitzins in Abhängigkeit der Arbeitslosenquote gesenkt
    Leitzinsaenderung = Leitzinsaenderung + max(-0.01,0.1 * (Arbeitslosentoleranzquote - Arbeitslosenquote) + 0.001); 
    
    % Inflation mit dem Leitzins an die Zielinflation anpassen
    Leitzinsaenderung = Leitzinsaenderung + 0.01 * (Inflation - (Inflationsziel + Inflationstoleranz));
        
    if Leitzins < 0.01 && Leitzinsaenderung < -0.001
        Leitzins = Leitzins - 0.001;
    else        
        Leitzins = Leitzins + Leitzinsaenderung;
    end   
    
LeitzinsOut = Leitzins;
MindestreservesatzOut = Mindestreservesatz;
MaximaleNotenbankGeldmengeOut = MaximaleNotenbankGeldmenge;
